simulink model "NavFilterTestHarness24"  (R2024b)
settings: Solver=FixedStepDiscrete  StartTime=startTime  StopTime=endTime  FixedStep=0.001  RelTol=1e-3  EnableMultiTasking=on
undefined symbols (not defined in the file): accel, ADSframe, ADStime, alignTime, angRate, ATTframe, CourseDeg, EAS2TAS, GndSpd, GPSframe, GPStime, Hgt, IMUframe, IMUtime, LatDeg, LngDeg, MagBiasX, MagBiasY, MagBiasZ, MAGframe, MAGtime, MagX, MagY, MagZ, msecHgtDelay, msecMagDelay, msecPosDelay, msecTasDelay, msecVelDelay, Pitch, Roll, Veas, VelD, Yaw
libraries: simulink x9, simulink_need_slupdate x2
(part 5 of 5)

== matlab function NavFilterTestHarness24/InertialNavFilter/Fuse True Airspeed Measurements ==
  data: states input; P input; FuseData input; VtasMea input; nextStates output; nextP output; innovation output; StatesAtMeasTime input; varInnov output; useAirspeed input
%#codegen
function [...
    nextStates, ... % state vector after fusion of measurements
    nextP, ... % state covariance matrix after fusion of corrections
    innovation, ... % True airspeed innovations (m/s)
    varInnov] ... % True airspeed innovation variance (m/s)^2
    = FuseAirspeed( ...
    states, ... % predicted states from the INS (q0, ... , q3, VelN,E,D, PosN,E,D, WindN,E, P0, camera roll pitch yaw misalignment)
    P, ... % predicted covariance
    FuseData, ... % Boolean to initiate fusion of airspeed measurements
    VtasMea, ... % true airspeed measurement (m/s)
    StatesAtMeasTime, ... % states at time of airspeed measurement
    useAirspeed) % Boolean to indicate that a airspeed sensor is being used

% define arrays used to calculate intermediate result in covariance
% update
KH  = single(zeros(24,24));
KHP = single(zeros(24,24));

% initialise innovation
innovation = single(0);

% initialise innovation variance vector (for data analysis only)
varInnov = single(0);

% Airspeed measurement error variance (m/s)^2.
R_TAS = single(2.0);

% Copy required states to local variable names
vn = single(StatesAtMeasTime(5));
ve = single(StatesAtMeasTime(6));
vd = single(StatesAtMeasTime(7));
vwn = single(StatesAtMeasTime(17));
vwe = single(StatesAtMeasTime(18));

% Calculate the airspeed prediction
VtasPred = sqrt((ve - vwe)^2 + (vn - vwn)^2 + vd^2);
% Need to check that it is flying before fusing airspeed data due to
if (useAirspeed && FuseData && (VtasPred > 1.0) && VtasMea > 8.0)
    % Sequential fusion of XYZ components
    
    % Calculate observation jacobians
    SH_TAS = single(zeros(3,1));
    SH_TAS(1) = 1/VtasPred;
    SH_TAS(2) = (SH_TAS(1)*(2*ve - 2*vwe))/2;
    SH_TAS(3) = (SH_TAS(1)*(2*vn - 2*vwn))/2;
    
    H_TAS = single(zeros(1,24));
    H_TAS(1,5) = SH_TAS(3);
    H_TAS(1,6) = SH_TAS(2);
    H_TAS(1,7) = vd*SH_TAS(1);
    H_TAS(1,17) = -SH_TAS(3);
    H_TAS(1,18) = -SH_TAS(2);
    
    SK_TAS = 1/(R_TAS + SH_TAS(3)*(P(5,5)*SH_TAS(3) + P(6,5)*SH_TAS(2) - P(17,5)*SH_TAS(3) - P(18,5)*SH_TAS(2) + P(7,5)*vd*SH_TAS(1)) + SH_TAS(2)*(P(5,6)*SH_TAS(3) + P(6,6)*SH_TAS(2) - P(17,6)*SH_TAS(3) - P(18,6)*SH_TAS(2) + P(7,6)*vd*SH_TAS(1)) - SH_TAS(3)*(P(5,17)*SH_TAS(3) + P(6,17)*SH_TAS(2) - P(17,17)*SH_TAS(3) - P(18,17)*SH_TAS(2) + P(7,17)*vd*SH_TAS(1)) - SH_TAS(2)*(P(5,18)*SH_TAS(3) + P(6,18)*SH_TAS(2) - P(17,18)*SH_TAS(3) - P(18,18)*SH_TAS(2) + P(7,18)*vd*SH_TAS(1)) + vd*SH_TAS(1)*(P(5,7)*SH_TAS(3) + P(6,7)*SH_TAS(2) - P(17,7)*SH_TAS(3) - P(18,7)*SH_TAS(2) + P(7,7)*vd*SH_TAS(1)));
    
    K_TAS = single(zeros(24,1));
    K_TAS(1,1) = SK_TAS*(P(1,5)*SH_TAS(3) - P(1,17)*SH_TAS(3) + P(1,6)*SH_TAS(2) - P(1,18)*SH_TAS(2) + P(1,7)*vd*SH_TAS(1));
    K_TAS(2,1) = SK_TAS*(P(2,5)*SH_TAS(3) - P(2,17)*SH_TAS(3) + P(2,6)*SH_TAS(2) - P(2,18)*SH_TAS(2) + P(2,7)*vd*SH_TAS(1));
    K_TAS(3,1) = SK_TAS*(P(3,5)*SH_TAS(3) - P(3,17)*SH_TAS(3) + P(3,6)*SH_TAS(2) - P(3,18)*SH_TAS(2) + P(3,7)*vd*SH_TAS(1));
    K_TAS(4,1) = SK_TAS*(P(4,5)*SH_TAS(3) - P(4,17)*SH_TAS(3) + P(4,6)*SH_TAS(2) - P(4,18)*SH_TAS(2) + P(4,7)*vd*SH_TAS(1));
    K_TAS(5,1) = SK_TAS*(P(5,5)*SH_TAS(3) - P(5,17)*SH_TAS(3) + P(5,6)*SH_TAS(2) - P(5,18)*SH_TAS(2) + P(5,7)*vd*SH_TAS(1));
    K_TAS(6,1) = SK_TAS*(P(6,5)*SH_TAS(3) - P(6,17)*SH_TAS(3) + P(6,6)*SH_TAS(2) - P(6,18)*SH_TAS(2) + P(6,7)*vd*SH_TAS(1));
    K_TAS(7,1) = SK_TAS*(P(7,5)*SH_TAS(3) - P(7,17)*SH_TAS(3) + P(7,6)*SH_TAS(2) - P(7,18)*SH_TAS(2) + P(7,7)*vd*SH_TAS(1));
    K_TAS(8,1) = SK_TAS*(P(8,5)*SH_TAS(3) - P(8,17)*SH_TAS(3) + P(8,6)*SH_TAS(2) - P(8,18)*SH_TAS(2) + P(8,7)*vd*SH_TAS(1));
    K_TAS(9,1) = SK_TAS*(P(9,5)*SH_TAS(3) - P(9,17)*SH_TAS(3) + P(9,6)*SH_TAS(2) - P(9,18)*SH_TAS(2) + P(9,7)*vd*SH_TAS(1));
    K_TAS(10,1) = SK_TAS*(P(10,5)*SH_TAS(3) - P(10,17)*SH_TAS(3) + P(10,6)*SH_TAS(2) - P(10,18)*SH_TAS(2) + P(10,7)*vd*SH_TAS(1));
    K_TAS(11,1) = SK_TAS*(P(11,5)*SH_TAS(3) - P(11,17)*SH_TAS(3) + P(11,6)*SH_TAS(2) - P(11,18)*SH_TAS(2) + P(11,7)*vd*SH_TAS(1));
    K_TAS(12,1) = SK_TAS*(P(12,5)*SH_TAS(3) - P(12,17)*SH_TAS(3) + P(12,6)*SH_TAS(2) - P(12,18)*SH_TAS(2) + P(12,7)*vd*SH_TAS(1));
    K_TAS(13,1) = SK_TAS*(P(13,5)*SH_TAS(3) - P(13,17)*SH_TAS(3) + P(13,6)*SH_TAS(2) - P(13,18)*SH_TAS(2) + P(13,7)*vd*SH_TAS(1));
    K_TAS(14,1) = SK_TAS*(P(14,5)*SH_TAS(3) - P(14,17)*SH_TAS(3) + P(14,6)*SH_TAS(2) - P(14,18)*SH_TAS(2) + P(14,7)*vd*SH_TAS(1));
    K_TAS(15,1) = SK_TAS*(P(15,5)*SH_TAS(3) - P(15,17)*SH_TAS(3) + P(15,6)*SH_TAS(2) - P(15,18)*SH_TAS(2) + P(15,7)*vd*SH_TAS(1));
    K_TAS(16,1) = SK_TAS*(P(16,5)*SH_TAS(3) - P(16,17)*SH_TAS(3) + P(16,6)*SH_TAS(2) - P(16,18)*SH_TAS(2) + P(16,7)*vd*SH_TAS(1));
    K_TAS(17,1) = SK_TAS*(P(17,5)*SH_TAS(3) - P(17,17)*SH_TAS(3) + P(17,6)*SH_TAS(2) - P(17,18)*SH_TAS(2) + P(17,7)*vd*SH_TAS(1));
    K_TAS(18,1) = SK_TAS*(P(18,5)*SH_TAS(3) - P(18,17)*SH_TAS(3) + P(18,6)*SH_TAS(2) - P(18,18)*SH_TAS(2) + P(18,7)*vd*SH_TAS(1));
    K_TAS(19,1) = SK_TAS*(P(19,5)*SH_TAS(3) - P(19,17)*SH_TAS(3) + P(19,6)*SH_TAS(2) - P(19,18)*SH_TAS(2) + P(19,7)*vd*SH_TAS(1));
    K_TAS(20,1) = SK_TAS*(P(20,5)*SH_TAS(3) - P(20,17)*SH_TAS(3) + P(20,6)*SH_TAS(2) - P(20,18)*SH_TAS(2) + P(20,7)*vd*SH_TAS(1));
    K_TAS(21,1) = SK_TAS*(P(21,5)*SH_TAS(3) - P(21,17)*SH_TAS(3) + P(21,6)*SH_TAS(2) - P(21,18)*SH_TAS(2) + P(21,7)*vd*SH_TAS(1));
    K_TAS(22,1) = SK_TAS*(P(22,5)*SH_TAS(3) - P(22,17)*SH_TAS(3) + P(22,6)*SH_TAS(2) - P(22,18)*SH_TAS(2) + P(22,7)*vd*SH_TAS(1));
    K_TAS(23,1) = SK_TAS*(P(23,5)*SH_TAS(3) - P(23,17)*SH_TAS(3) + P(23,6)*SH_TAS(2) - P(23,18)*SH_TAS(2) + P(23,7)*vd*SH_TAS(1));
    K_TAS(24,1) = SK_TAS*(P(24,5)*SH_TAS(3) - P(24,17)*SH_TAS(3) + P(24,6)*SH_TAS(2) - P(24,18)*SH_TAS(2) + P(24,7)*vd*SH_TAS(1));
    
    % calculate the innovation variance (for data logging only)
    varInnov = 1/SK_TAS;
    
    % correct the states
    innovation = VtasPred - VtasMea;
    % Check the innovation for consistencey and don't fuse if > 5 Sigma
    if (SK_TAS * innovation^2) < 25.0
        xk = K_TAS * innovation;
        states = states - xk;
        % Normalise the quaternion states
        quatMag = sqrt(states(1)^2 + states(2)^2 + states(3)^2 + states(4)^2);
        if (quatMag > 1e-12)
            states(1:4) = states(1:4) / quatMag;
        end
        % correct the covariance P = (I - K*H)*P
        % take advantage of the empty columns in H_TAS to reduce the
        % number of operations
        for i = 1:24
            for j = 5:7
                KH(i,j) = K_TAS(i)*H_TAS(j);
            end
            for j = 17:18
                KH(i,j) = K_TAS(i)*H_TAS(j);
            end
        end
        for i = 1:24
            for j = 1:24
                for k = 5:7
                    KHP(i,j) = KHP(i,j) + KH(i,k)*P(k,j);
                end
                for k = 17:18
                    KHP(i,j) = KHP(i,j) + KH(i,k)*P(k,j);
                end
            end
        end
        P = P - KHP;
    end
end

% Set output for states and covariance
nextP = P;
nextStates   = states;

end

== matlab function NavFilterTestHarness24/InertialNavFilter/Recall States2 ==
  data: fuseData output; statesStore input; msecStore input; msecDelay input; statesOut output; states input; time input; newDataArrived input
%#codegen
function [fuseData,statesOut]    = RecallStates2(statesStore,msecStore,msecDelay,states,time,newDataArrived)
persistent statesForFusion;
if isempty(statesForFusion)
    statesForFusion = single(zeros(24,1));
end
bestTimeDelta = int32(msecDelay);
bestStoreIndex = 1;
if newDataArrived
    for storeIndex=1:50
        timeDelta = (int32(time*1000) - int32(msecDelay)) - int32(msecStore(storeIndex));
        if (timeDelta < 0)
            timeDelta = -timeDelta;
        end
        if (timeDelta < bestTimeDelta)
            bestStoreIndex = storeIndex;
            bestTimeDelta = timeDelta;
        end
    end
    if (bestTimeDelta < msecDelay) % only output stored state if time accuracy better than just outputtting current states
        for i=1:24
            statesForFusion(i) = statesStore(i,bestStoreIndex);
        end
    else % otherwise output current state
        for i=1:24
            statesForFusion(i) = states(i);
        end
    end
end
statesOut = statesForFusion;
fuseData = newDataArrived;
end

== matlab function NavFilterTestHarness24/InertialNavFilter/Calc Initial Parameters/Embedded MATLAB Function ==
  data: earthRateNED output; covariance output; latDeg input
function [earthRateNED, covariance] = calculateInitialData(latDeg)
%#codegen

% degrees to to radians conversion
deg2rad = single(pi/180);

% Define the initial Euler angle covariance (Phi, Theta, Psi)
InitialEulerCovariance  = single([(1.0*pi/180); (1.0*pi/180); (10.0*pi/180)].^2);

% Define the transformation vector from a 321 sequence Euler rotation vector to a q0,...,q3 quaternion vector
% linearised around a level orientation (roll,pitch = 0,0)
J_eul2quat = ...
    single([[ 0.0, 0.0, 0.0]; ...
    [ 0.5, 0.0, 0.0]; ...
    [ 0.0, 0.5, 0.0]; ...
    [ 0.0, 0.0, 0.5]]);

% Form the covariance matrix for the intial Euler angle coordinates
angleCov = diag(InitialEulerCovariance);

% Transform the Euler angle covariances into the equivalent quaternion covariances
quatCov = J_eul2quat*angleCov*transpose(J_eul2quat);

% define the state covariances with the exception of the quaternion covariances
Sigma_vel_NE = single(0.7); % 1 sigma uncertainty in horizontal velocity components
Sigma_vel_D  = single(0.7); % 1 sigma uncertainty in vertical velocity
Sigma_pos_NE = single(15); % 1 sigma uncertainty in horizontal position components
Sigma_pos_D  = single(5.0); % 1 sigma uncertainty in vertical position
Sigma_dAng   = single(1/10*pi/180*0.02); % 1 Sigma uncertainty in delta angle bias
Sigma_dVel   = single(0.1*0.02); % 1 Sigma uncertainty in delta velocity bias
Sigma_wind   = single(8);
Sigma_MagNED = single(20);
Sigma_MagXYZ = single(20);
covariance   = single(diag([0;0;0;0;Sigma_vel_NE*[1;1];Sigma_vel_D;Sigma_pos_NE*[1;1];Sigma_pos_D;Sigma_dAng*[1;1;1];Sigma_dVel*[1;1;1];Sigma_wind*[1;1];Sigma_MagNED*[1;1;1];Sigma_MagXYZ*[1;1;1]].^2));

% Add the quaternion covariances
covariance(1:4,1:4) = quatCov;

%Define Earth rotation vector in the NED navigation frame
earthRateECEF = single([0; 0; 7.2921e-005]);
earthRateNED  = ...
    single([cos(latDeg*deg2rad)*earthRateECEF(3); ...
    0; ...
    -sin(latDeg*deg2rad)*earthRateECEF(3)]);

== matlab function NavFilterTestHarness24/InertialNavFilter/Recall States3 ==
  data: fuseData output; statesStore input; msecStore input; msecDelay input; statesOut output; states input; time input; newDataArrived input
%#codegen
function [fuseData,statesOut]    = RecallStates3(statesStore,msecStore,msecDelay,states,time,newDataArrived)
persistent statesForFusion;
if isempty(statesForFusion)
    statesForFusion = single(zeros(24,1));
end
bestTimeDelta = int32(msecDelay);
bestStoreIndex = 1;
if newDataArrived
    for storeIndex=1:50
        timeDelta = (int32(time*1000) - int32(msecDelay)) - int32(msecStore(storeIndex));
        if (timeDelta < 0)
            timeDelta = -timeDelta;
        end
        if (timeDelta < bestTimeDelta)
            bestStoreIndex = storeIndex;
            bestTimeDelta = timeDelta;
        end
    end
    if (bestTimeDelta < msecDelay) % only output stored state if time accuracy better than just outputtting current states
        for i=1:24
            statesForFusion(i) = statesStore(i,bestStoreIndex);
        end
    else % otherwise output current state
        for i=1:24
            statesForFusion(i) = states(i);
        end
    end
end
statesOut = statesForFusion;
fuseData = newDataArrived;
end
